simulink model "ProcessFlowRateModel_symbiotic"  (Simulink 7.9)
settings: Solver=VariableStepDiscrete  StartTime=0.0  StopTime=5000  RelTol=1e-3
libraries: simeventslib x11
settings Model: Creator=tsprock3  LastModifiedBy=tsprock3
settings DebuggingCC: SimStateOlderReleaseMsg=warning

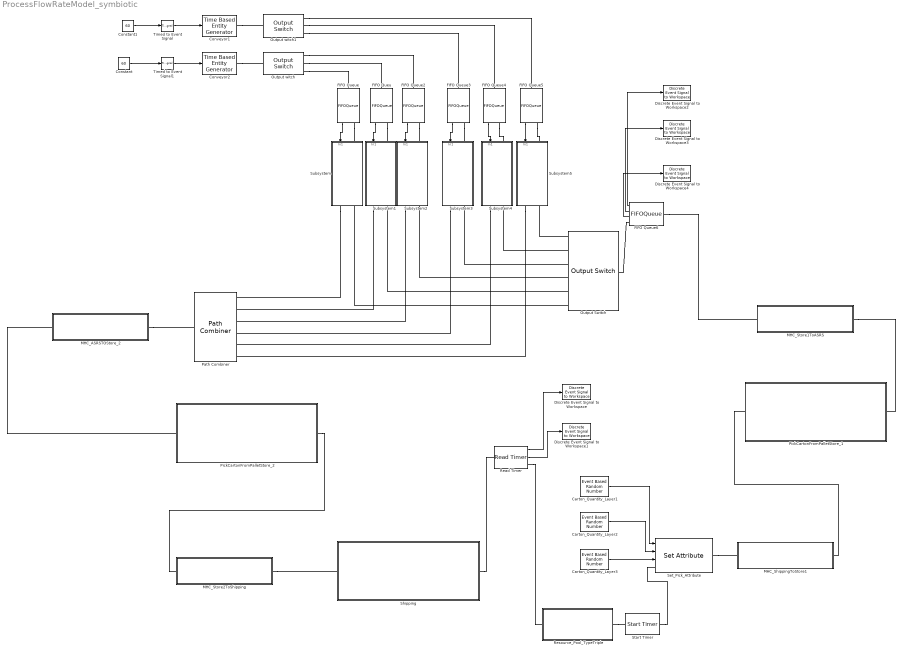
== system ProcessFlowRateModel_symbiotic ==
  Carton_Quantity_Layer1 : EventBasedRandomNumber  Distribution=Discrete uniform  minUnid=17  maxUnid=23  numValueUnid=7  valueVecDisc=[1 2 3]  probVecDisc=[0.5 0.35 0.15]  Seed=35621
  Carton_Quantity_Layer2 : EventBasedRandomNumber  Distribution=Discrete uniform  minUnid=55  maxUnid=65  numValueUnid=11  valueVecDisc=[1 2 3]  probVecDisc=[0.5 0.35 0.15]  Seed=38838
  Carton_Quantity_Layer3 : EventBasedRandomNumber  Distribution=Discrete uniform  minUnid=17  maxUnid=23  numValueUnid=7  valueVecDisc=[1 2 3]  probVecDisc=[0.5 0.35 0.15]  Seed=42055
  Constant : Constant  Value=60
  Constant1 : Constant  Value=60
  Conveyor1 : TimeBasedEntityGenerator  GenerateEntitiesUpon=Intergeneration time from port t
  Conveyor2 : TimeBasedEntityGenerator  GenerateEntitiesUpon=Intergeneration time from port t
  Discrete Event Signal to Workspace : simeventslib/SimEvents Sinks/Discrete Event Signal to Workspace  VariableName=elapsedtime  SaveFormat=Structure With Time  isMonitorOnly=off  isRecordIC=off
  Discrete Event Signal to Workspace1 : simeventslib/SimEvents Sinks/Discrete Event Signal to Workspace  VariableName=avg  SaveFormat=Structure With Time  isMonitorOnly=off  isRecordIC=off
  Discrete Event Signal to Workspace2 : simeventslib/SimEvents Sinks/Discrete Event Signal to Workspace  VariableName=serviced_qty  SaveFormat=Structure With Time  isMonitorOnly=off  isRecordIC=off
  Discrete Event Signal to Workspace3 : simeventslib/SimEvents Sinks/Discrete Event Signal to Workspace  VariableName=num_wait  SaveFormat=Structure With Time  isMonitorOnly=off  isRecordIC=off
  Discrete Event Signal to Workspace4 : simeventslib/SimEvents Sinks/Discrete Event Signal to Workspace  VariableName=avg_wait  SaveFormat=Structure With Time  isMonitorOnly=off  isRecordIC=off
  FIFO Queu : FIFOQueue  Capacity=1  StatNumberInBlock=on
      settings: OutputPortMap=o1
  FIFO Queue{,2..5} (5 alike) : FIFOQueue  Capacity=1  StatNumberInBlock=on
      settings: OutputPortMap=o1
  FIFO Queue6 : FIFOQueue  StatNumberDeparted=on  StatNumberInBlock=on  StatAverageWait=on
      settings: OutputPortMap=o0,o1,o2
  MHC_ASRSTOStore_2 : Subsystem
  MHC_ShippingToStore1 : Subsystem
  MHC_Store1ToASRS : Subsystem
  MHC_Store2ToShipping : Subsystem
  Output Switch : OutputSwitch  NumberOutputPorts=6
  Output witch : OutputSwitch  SwitchingCriterion=Round robin
  Output witch1 : OutputSwitch  SwitchingCriterion=Round robin
  Path Combiner : PathCombiner  NumberInputPorts=6
  PickCartonFromPalletStore_1 : Subsystem
  PickCartonFromPalletStore_2 : Subsystem
  Read Timer : ReadTimer  StatTimeElapsed=on  StatAverageTimeElapsed=on
      settings: OutputPortMap=o2,o3
  Resource_Pool_TypeTriple : Subsystem  mask{Quantity=33}
      mask prompts: Quantity "How many entities in resource pool?"
  Set_Pick_Attribute : SetAttribute  AttributeName=Carton_Quantity_Layer1|Carton_Quantity_Layer2|Carton_Quantity_Layer3  AttributeFrom=Signal port|Signal port|Signal port  AttributeValue=1|1|1  AttributeTreatAsVector=1|1|1  EvaluatedAttributeValue={[];[];[]}
      settings: InputPortMap=u0,u1,u2
  Shipping : Subsystem
  Start Timer : StartTimer  TimerStartedOption=Restart
  Subsystem : Subsystem
  Subsystem1 : Subsystem
  Subsystem2 : Subsystem
  Subsystem3 : Subsystem
  Subsystem4 : Subsystem
  Subsystem5 : Subsystem
  Timed to Event Signal : TimedToEventSignal
  Timed to Event Signal1 : TimedToEventSignal
  wires:
  Read Timer/1 -> Discrete Event Signal to Workspace/1
  Read Timer/2 -> Discrete Event Signal to Workspace1/1
  Carton_Quantity_Layer1/1 -> Set_Pick_Attribute/1
  Carton_Quantity_Layer2/1 -> Set_Pick_Attribute/2
  Carton_Quantity_Layer3/1 -> Set_Pick_Attribute/3
  FIFO Queue6/3 -> Discrete Event Signal to Workspace4/1
  FIFO Queue6/2 -> Discrete Event Signal to Workspace3/1
  FIFO Queue6/1 -> Discrete Event Signal to Workspace2/1
  Constant1/1 -> Timed to Event Signal/1
  Timed to Event Signal/1 -> Conveyor1/1
  Constant/1 -> Timed to Event Signal1/1
  Timed to Event Signal1/1 -> Conveyor2/1
  FIFO Queue/1 -> Subsystem/1(In1)
  FIFO Queu/1 -> Subsystem1/1(In1)
  FIFO Queue2/1 -> Subsystem2/1(In1)
  FIFO Queue3/1 -> Subsystem3/1(In1)
  FIFO Queue4/1 -> Subsystem4/1(In1)
  FIFO Queue5/1 -> Subsystem5/1(In1)
  connections:
  Set_Pick_Attribute/RConn1 -- MHC_ShippingToStore1/LConn1
  MHC_Store2ToShipping/RConn1 -- Shipping/LConn1
  MHC_ShippingToStore1/RConn1 -- PickCartonFromPalletStore_1/LConn1
  MHC_Store1ToASRS/LConn1 -- PickCartonFromPalletStore_1/RConn1
  PickCartonFromPalletStore_2/RConn1 -- MHC_Store2ToShipping/LConn1
  MHC_ASRSTOStore_2/RConn1 -- PickCartonFromPalletStore_2/LConn1
  Conveyor2/RConn1 -- Output witch/LConn1
  Output witch/RConn3 -- FIFO Queue/LConn1
  Output witch/RConn2 -- FIFO Queu/LConn1
  Output witch/RConn1 -- FIFO Queue2/LConn1
  Conveyor1/RConn1 -- Output witch1/LConn1
  Output witch1/RConn1 -- FIFO Queue5/LConn1
  Output witch1/RConn2 -- FIFO Queue4/LConn1
  Output witch1/RConn3 -- FIFO Queue3/LConn1
  FIFO Queue6/LConn1 -- MHC_Store1ToASRS/RConn1
  Shipping/RConn1 -- Read Timer/LConn1
  Resource_Pool_TypeTriple/LConn1 -- Start Timer/LConn1
  Start Timer/RConn1 -- Set_Pick_Attribute/LConn1
  Read Timer/RConn1 -- Resource_Pool_TypeTriple/RConn1
  FIFO Queue/RConn1 -- Subsystem/LConn1
  FIFO Queu/RConn1 -- Subsystem1/LConn1
  FIFO Queue2/RConn1 -- Subsystem2/LConn1
  FIFO Queue3/RConn1 -- Subsystem3/LConn1
  FIFO Queue4/RConn1 -- Subsystem4/LConn1
  FIFO Queue5/RConn1 -- Subsystem5/LConn1
  MHC_ASRSTOStore_2/LConn1 -- Path Combiner/RConn1
  Output Switch/LConn1 -- FIFO Queue6/RConn1
  Output Switch/RConn1 -- Subsystem5/RConn2
  Output Switch/RConn2 -- Subsystem4/RConn2
  Output Switch/RConn3 -- Subsystem3/RConn2
  Output Switch/RConn4 -- Subsystem2/RConn2
  Output Switch/RConn5 -- Subsystem1/RConn2
  Output Switch/RConn6 -- Subsystem/RConn2
  Subsystem/RConn1 -- Path Combiner/LConn1
  Subsystem1/RConn1 -- Path Combiner/LConn2
  Subsystem2/RConn1 -- Path Combiner/LConn3
  Subsystem3/RConn1 -- Path Combiner/LConn4
  Subsystem4/RConn1 -- Path Combiner/LConn5
  Subsystem5/RConn1 -- Path Combiner/LConn6

== system ProcessFlowRateModel_symbiotic/MHC_ASRSTOStore_2 ==
  note: This level provides an interface to access the Transportation_Channel block variant. The interface provides a method to
      | bring shipments in and route shipments out, as well as a consistent method to add ports to realize that interface
  IN_Shipment : PathCombiner  NumberInputPorts=1
  OUT_Shipment : OutputSwitch  NumberOutputPorts=1  AttributeName=Customer
  Transportation_Channel : Subsystem
  IN_Shipment_1 : PMIOPort  Port=1  Side=Left
  OUT_Shipment_1 : PMIOPort  Port=2  Side=Right
  connections:
  IN_Shipment/RConn1 -- Transportation_Channel/LConn1
  Transportation_Channel/RConn1 -- OUT_Shipment/LConn1
  IN_Shipment_1/RConn1 -- IN_Shipment/LConn1
  OUT_Shipment/RConn1 -- OUT_Shipment_1/RConn1

== system ProcessFlowRateModel_symbiotic/MHC_ShippingToStore1 ==
  note: This level provides an interface to access the Transportation_Channel block variant. The interface provides a method to
      | bring shipments in and route shipments out, as well as a consistent method to add ports to realize that interface
  IN_Shipment : PathCombiner  NumberInputPorts=1
  OUT_Shipment : OutputSwitch  NumberOutputPorts=1  AttributeName=Customer
  Transportation_Channel : Subsystem
  IN_Shipment_1 : PMIOPort  Port=1  Side=Left
  OUT_Shipment_1 : PMIOPort  Port=2  Side=Right
  connections:
  IN_Shipment/RConn1 -- Transportation_Channel/LConn1
  Transportation_Channel/RConn1 -- OUT_Shipment/LConn1
  IN_Shipment_1/RConn1 -- IN_Shipment/LConn1
  OUT_Shipment/RConn1 -- OUT_Shipment_1/RConn1

== system ProcessFlowRateModel_symbiotic/MHC_Store1ToASRS ==
  note: This level provides an interface to access the Transportation_Channel block variant. The interface provides a method to
      | bring shipments in and route shipments out, as well as a consistent method to add ports to realize that interface
  IN_Shipment : PathCombiner  NumberInputPorts=1
  OUT_Shipment : OutputSwitch  NumberOutputPorts=1  AttributeName=Customer
  Transportation_Channel : Subsystem
  IN_Shipment_1 : PMIOPort  Port=1  Side=Left
  OUT_Shipment_1 : PMIOPort  Port=2  Side=Right
  connections:
  IN_Shipment/RConn1 -- Transportation_Channel/LConn1
  Transportation_Channel/RConn1 -- OUT_Shipment/LConn1
  IN_Shipment_1/RConn1 -- IN_Shipment/LConn1
  OUT_Shipment/RConn1 -- OUT_Shipment_1/RConn1

== system ProcessFlowRateModel_symbiotic/MHC_Store2ToShipping ==
  note: This level provides an interface to access the Transportation_Channel block variant. The interface provides a method to
      | bring shipments in and route shipments out, as well as a consistent method to add ports to realize that interface
  IN_Shipment : PathCombiner  NumberInputPorts=1
  OUT_Shipment : OutputSwitch  NumberOutputPorts=1  AttributeName=Customer
  Transportation_Channel : Subsystem
  IN_Shipment_1 : PMIOPort  Port=1  Side=Left
  OUT_Shipment_1 : PMIOPort  Port=2  Side=Right
  connections:
  IN_Shipment/RConn1 -- Transportation_Channel/LConn1
  Transportation_Channel/RConn1 -- OUT_Shipment/LConn1
  IN_Shipment_1/RConn1 -- IN_Shipment/LConn1
  OUT_Shipment/RConn1 -- OUT_Shipment_1/RConn1

== system ProcessFlowRateModel_symbiotic/PickCartonFromPalletStore_1 ==
  IN_Job : PathCombiner  NumberInputPorts=1
  OUT_Job : OutputSwitch  NumberOutputPorts=1  SwitchingCriterion=Equiprobable  InitialSeed=9514
  Workstation : Subsystem
  IN_Job_1 : PMIOPort  Port=1  Side=Left
  OUT_Job_1 : PMIOPort  Port=2  Side=Right
  connections:
  IN_Job/RConn1 -- Workstation/LConn1
  Workstation/RConn1 -- OUT_Job/LConn1
  IN_Job_1/RConn1 -- IN_Job/LConn1
  OUT_Job/RConn1 -- OUT_Job_1/RConn1

== system ProcessFlowRateModel_symbiotic/PickCartonFromPalletStore_2 ==
  IN_Job : PathCombiner  NumberInputPorts=1
  OUT_Job : OutputSwitch  NumberOutputPorts=1  SwitchingCriterion=Equiprobable  InitialSeed=12731
  Workstation : Subsystem
  IN_Job_1 : PMIOPort  Port=1  Side=Left
  OUT_Job_1 : PMIOPort  Port=2  Side=Right
  connections:
  IN_Job/RConn1 -- Workstation/LConn1
  Workstation/RConn1 -- OUT_Job/LConn1
  IN_Job_1/RConn1 -- IN_Job/LConn1
  OUT_Job/RConn1 -- OUT_Job_1/RConn1

== system ProcessFlowRateModel_symbiotic/Resource_Pool_TypeTriple ==
  Event-Based Entity Generator : EventBasedEntityGenerator  GenerateEntitiesUpon=Function call from port fcn
  FIFO Queue : FIFOQueue  Capacity=inf
  FIFO Queue1 : FIFOQueue  Capacity=inf
  Path Combiner : PathCombiner  NumberInputPorts=2
  Release Gate : ReleaseGate  OpenGateUpon=Function call from port fcn
  Time-Based Function-Call Generator : TimeBasedFunctionCallGenerator  EventGenerationMode=Only at simulation start  NumberOfEventsPerPeriod=Quantity
  Time-Based Function-Call Generator1 : TimeBasedFunctionCallGenerator
  Acquire : PMIOPort  Port=1  Side=Left
  Return : PMIOPort  Port=2  Side=Right
  wires:
  Time-Based Function-Call Generator/1 -> Event-Based Entity Generator/1
  Time-Based Function-Call Generator1/1 -> Release Gate/1
  connections:
  Path Combiner/RConn1 -- FIFO Queue/LConn1
  Return/RConn1 -- Path Combiner/LConn2
  Acquire/RConn1 -- FIFO Queue/RConn1
  Event-Based Entity Generator/RConn1 -- FIFO Queue1/LConn1
  Release Gate/RConn1 -- Path Combiner/LConn1
  FIFO Queue1/RConn1 -- Release Gate/LConn1

== system ProcessFlowRateModel_symbiotic/Shipping ==
  IN_Job : PathCombiner  NumberInputPorts=1
  OUT_Job : OutputSwitch  NumberOutputPorts=1  SwitchingCriterion=Equiprobable  InitialSeed=15948
  Workstation : Subsystem
  IN_Job_1 : PMIOPort  Port=1  Side=Left
  OUT_Job_1 : PMIOPort  Port=2  Side=Right
  connections:
  IN_Job/RConn1 -- Workstation/LConn1
  Workstation/RConn1 -- OUT_Job/LConn1
  IN_Job_1/RConn1 -- IN_Job/LConn1
  OUT_Job/RConn1 -- OUT_Job_1/RConn1

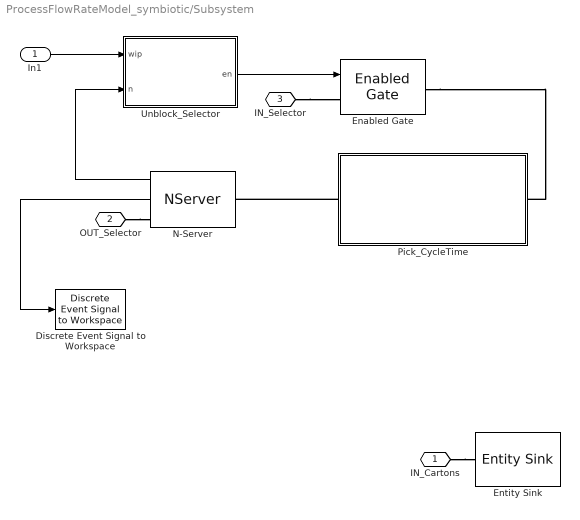
== system ProcessFlowRateModel_symbiotic/Subsystem ==
  In1 : Inport
  Discrete Event Signal to Workspace : simeventslib/SimEvents Sinks/Discrete Event Signal to Workspace  VariableName=utilization  SaveFormat=Structure With Time  isMonitorOnly=off  isRecordIC=off
  Enabled Gate : EnabledGate
  Entity Sink : EntitySink
  N-Server : NServer  NumberOfServers=1  ServiceTimeFrom=Attribute  ServiceTime=0  AttributeName=PickCycleTime  StatNumberInBlock=on  StatUtilization=on
      settings: OutputPortMap=o1,o5
  Pick_CycleTime : Subsystem  mask{pickmean=5, pickstddev=0.25, traveltime=0, qty=60}
      mask prompts: pickmean "eachPickMean"; pickstddev "eachPickStdDev"; qty "carton_qty"
  Unblock_Selector : Truth Table  TreatAsAtomicUnit=on
  IN_Cartons : PMIOPort  Port=1  Side=Left
  OUT_Selector : PMIOPort  Port=2  Side=Right
  IN_Selector : PMIOPort  Port=3  Side=Right
  wires:
  N-Server/2 -> Discrete Event Signal to Workspace/1
  In1/1 -> Unblock_Selector/1(wip)
  N-Server/1 -> Unblock_Selector/2(n)
  Unblock_Selector/1(en) -> Enabled Gate/1
  connections:
  Enabled Gate/RConn1 -- Pick_CycleTime/LConn1
  Pick_CycleTime/RConn1 -- N-Server/LConn1
  IN_Cartons/RConn1 -- Entity Sink/LConn1
  IN_Selector/RConn1 -- Enabled Gate/LConn1
  OUT_Selector/RConn1 -- N-Server/RConn1

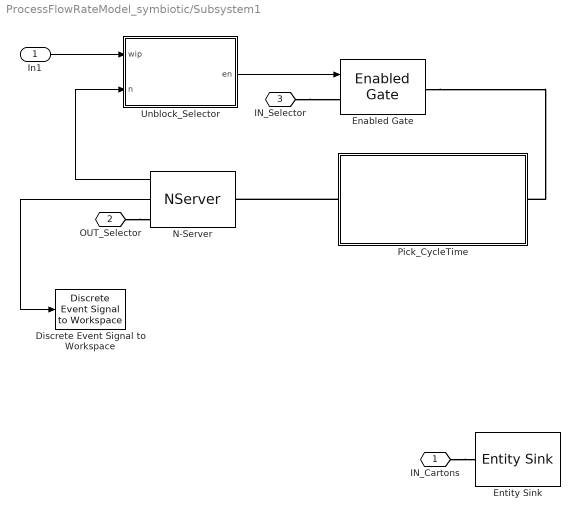
== system ProcessFlowRateModel_symbiotic/Subsystem1 ==
  In1 : Inport
  Discrete Event Signal to Workspace : simeventslib/SimEvents Sinks/Discrete Event Signal to Workspace  VariableName=utilization  SaveFormat=Structure With Time  isMonitorOnly=off  isRecordIC=off
  Enabled Gate : EnabledGate
  Entity Sink : EntitySink
  N-Server : NServer  NumberOfServers=1  ServiceTimeFrom=Attribute  ServiceTime=0  AttributeName=PickCycleTime  StatNumberInBlock=on  StatUtilization=on
      settings: OutputPortMap=o1,o5
  Pick_CycleTime : Subsystem  mask{pickmean=5, pickstddev=0.25, traveltime=0, qty=60}
      mask prompts: pickmean "eachPickMean"; pickstddev "eachPickStdDev"; qty "carton_qty"
  Unblock_Selector : Truth Table  TreatAsAtomicUnit=on
  IN_Cartons : PMIOPort  Port=1  Side=Left
  OUT_Selector : PMIOPort  Port=2  Side=Right
  IN_Selector : PMIOPort  Port=3  Side=Right
  wires:
  N-Server/2 -> Discrete Event Signal to Workspace/1
  In1/1 -> Unblock_Selector/1(wip)
  N-Server/1 -> Unblock_Selector/2(n)
  Unblock_Selector/1(en) -> Enabled Gate/1
  connections:
  Enabled Gate/RConn1 -- Pick_CycleTime/LConn1
  Pick_CycleTime/RConn1 -- N-Server/LConn1
  IN_Cartons/RConn1 -- Entity Sink/LConn1
  IN_Selector/RConn1 -- Enabled Gate/LConn1
  OUT_Selector/RConn1 -- N-Server/RConn1

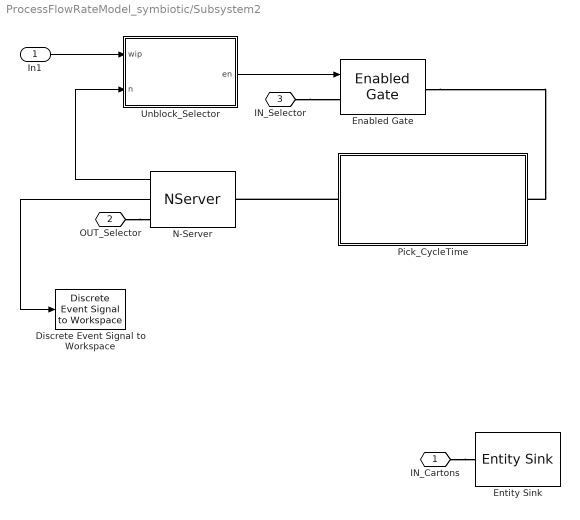
== system ProcessFlowRateModel_symbiotic/Subsystem2 ==
  In1 : Inport
  Discrete Event Signal to Workspace : simeventslib/SimEvents Sinks/Discrete Event Signal to Workspace  VariableName=utilization  SaveFormat=Structure With Time  isMonitorOnly=off  isRecordIC=off
  Enabled Gate : EnabledGate
  Entity Sink : EntitySink
  N-Server : NServer  NumberOfServers=1  ServiceTimeFrom=Attribute  ServiceTime=0  AttributeName=PickCycleTime  StatNumberInBlock=on  StatUtilization=on
      settings: OutputPortMap=o1,o5
  Pick_CycleTime : Subsystem  mask{pickmean=5, pickstddev=0.25, traveltime=0, qty=60}
      mask prompts: pickmean "eachPickMean"; pickstddev "eachPickStdDev"; qty "carton_qty"
  Unblock_Selector : Truth Table  TreatAsAtomicUnit=on
  IN_Cartons : PMIOPort  Port=1  Side=Left
  OUT_Selector : PMIOPort  Port=2  Side=Right
  IN_Selector : PMIOPort  Port=3  Side=Right
  wires:
  N-Server/2 -> Discrete Event Signal to Workspace/1
  In1/1 -> Unblock_Selector/1(wip)
  N-Server/1 -> Unblock_Selector/2(n)
  Unblock_Selector/1(en) -> Enabled Gate/1
  connections:
  Enabled Gate/RConn1 -- Pick_CycleTime/LConn1
  Pick_CycleTime/RConn1 -- N-Server/LConn1
  IN_Cartons/RConn1 -- Entity Sink/LConn1
  IN_Selector/RConn1 -- Enabled Gate/LConn1
  OUT_Selector/RConn1 -- N-Server/RConn1

== system ProcessFlowRateModel_symbiotic/Subsystem3 ==
  In1 : Inport
  Discrete Event Signal to Workspace : simeventslib/SimEvents Sinks/Discrete Event Signal to Workspace  VariableName=utilization  SaveFormat=Structure With Time  isMonitorOnly=off  isRecordIC=off
  Enabled Gate : EnabledGate
  Entity Sink : EntitySink
  N-Server : NServer  NumberOfServers=1  ServiceTimeFrom=Attribute  ServiceTime=0  AttributeName=PickCycleTime  StatNumberInBlock=on  StatUtilization=on
      settings: OutputPortMap=o1,o5
  Pick_CycleTime : Subsystem  mask{pickmean=5, pickstddev=0.25, traveltime=0, qty=60}
      mask prompts: pickmean "eachPickMean"; pickstddev "eachPickStdDev"; qty "carton_qty"
  Unblock_Selector : Truth Table  TreatAsAtomicUnit=on
  IN_Cartons : PMIOPort  Port=1  Side=Left
  OUT_Selector : PMIOPort  Port=2  Side=Right
  IN_Selector : PMIOPort  Port=3  Side=Right
  wires:
  N-Server/2 -> Discrete Event Signal to Workspace/1
  In1/1 -> Unblock_Selector/1(wip)
  N-Server/1 -> Unblock_Selector/2(n)
  Unblock_Selector/1(en) -> Enabled Gate/1
  connections:
  Enabled Gate/RConn1 -- Pick_CycleTime/LConn1
  Pick_CycleTime/RConn1 -- N-Server/LConn1
  IN_Cartons/RConn1 -- Entity Sink/LConn1
  IN_Selector/RConn1 -- Enabled Gate/LConn1
  OUT_Selector/RConn1 -- N-Server/RConn1

== system ProcessFlowRateModel_symbiotic/Subsystem4 ==
  In1 : Inport
  Discrete Event Signal to Workspace : simeventslib/SimEvents Sinks/Discrete Event Signal to Workspace  VariableName=utilization  SaveFormat=Structure With Time  isMonitorOnly=off  isRecordIC=off
  Enabled Gate : EnabledGate
  Entity Sink : EntitySink
  N-Server : NServer  NumberOfServers=1  ServiceTimeFrom=Attribute  ServiceTime=0  AttributeName=PickCycleTime  StatNumberInBlock=on  StatUtilization=on
      settings: OutputPortMap=o1,o5
  Pick_CycleTime : Subsystem  mask{pickmean=5, pickstddev=0.25, traveltime=0, qty=60}
      mask prompts: pickmean "eachPickMean"; pickstddev "eachPickStdDev"; qty "carton_qty"
  Unblock_Selector : Truth Table  TreatAsAtomicUnit=on
  IN_Cartons : PMIOPort  Port=1  Side=Left
  OUT_Selector : PMIOPort  Port=2  Side=Right
  IN_Selector : PMIOPort  Port=3  Side=Right
  wires:
  N-Server/2 -> Discrete Event Signal to Workspace/1
  In1/1 -> Unblock_Selector/1(wip)
  N-Server/1 -> Unblock_Selector/2(n)
  Unblock_Selector/1(en) -> Enabled Gate/1
  connections:
  Enabled Gate/RConn1 -- Pick_CycleTime/LConn1
  Pick_CycleTime/RConn1 -- N-Server/LConn1
  IN_Cartons/RConn1 -- Entity Sink/LConn1
  IN_Selector/RConn1 -- Enabled Gate/LConn1
  OUT_Selector/RConn1 -- N-Server/RConn1

== system ProcessFlowRateModel_symbiotic/Subsystem5 ==
  In1 : Inport
  Discrete Event Signal to Workspace : simeventslib/SimEvents Sinks/Discrete Event Signal to Workspace  VariableName=utilization  SaveFormat=Structure With Time  isMonitorOnly=off  isRecordIC=off
  Enabled Gate : EnabledGate
  Entity Sink : EntitySink
  N-Server : NServer  NumberOfServers=1  ServiceTimeFrom=Attribute  ServiceTime=0  AttributeName=PickCycleTime  StatNumberInBlock=on  StatUtilization=on
      settings: OutputPortMap=o1,o5
  Pick_CycleTime : Subsystem  mask{pickmean=5, pickstddev=0.25, traveltime=0, qty=60}
      mask prompts: pickmean "eachPickMean"; pickstddev "eachPickStdDev"; qty "carton_qty"
  Unblock_Selector : Truth Table  TreatAsAtomicUnit=on
  IN_Cartons : PMIOPort  Port=1  Side=Left
  OUT_Selector : PMIOPort  Port=2  Side=Right
  IN_Selector : PMIOPort  Port=3  Side=Right
  wires:
  N-Server/2 -> Discrete Event Signal to Workspace/1
  In1/1 -> Unblock_Selector/1(wip)
  N-Server/1 -> Unblock_Selector/2(n)
  Unblock_Selector/1(en) -> Enabled Gate/1
  connections:
  Enabled Gate/RConn1 -- Pick_CycleTime/LConn1
  Pick_CycleTime/RConn1 -- N-Server/LConn1
  IN_Cartons/RConn1 -- Entity Sink/LConn1
  IN_Selector/RConn1 -- Enabled Gate/LConn1
  OUT_Selector/RConn1 -- N-Server/RConn1

== system ProcessFlowRateModel_symbiotic/MHC_ASRSTOStore_2/Transportation_Channel ==
  FIFO Queue : FIFOQueue  Capacity=inf
  N-Server : NServer  NumberOfServers=inf  ServiceTime=10
  IN_Shipment : PMIOPort  Port=1  Side=Left
  OUT_Shipment : PMIOPort  Port=2  Side=Right
  connections:
  FIFO Queue/RConn1 -- N-Server/LConn1
  IN_Shipment/RConn1 -- FIFO Queue/LConn1
  OUT_Shipment/RConn1 -- N-Server/RConn1

== system ProcessFlowRateModel_symbiotic/MHC_ShippingToStore1/Transportation_Channel ==
  FIFO Queue : FIFOQueue  Capacity=inf
  N-Server : NServer  NumberOfServers=inf  ServiceTime=20
  IN_Shipment : PMIOPort  Port=1  Side=Left
  OUT_Shipment : PMIOPort  Port=2  Side=Right
  connections:
  FIFO Queue/RConn1 -- N-Server/LConn1
  IN_Shipment/RConn1 -- FIFO Queue/LConn1
  OUT_Shipment/RConn1 -- N-Server/RConn1

== system ProcessFlowRateModel_symbiotic/MHC_Store1ToASRS/Transportation_Channel ==
  FIFO Queue : FIFOQueue  Capacity=inf
  N-Server : NServer  NumberOfServers=inf  ServiceTime=10
  IN_Shipment : PMIOPort  Port=1  Side=Left
  OUT_Shipment : PMIOPort  Port=2  Side=Right
  connections:
  FIFO Queue/RConn1 -- N-Server/LConn1
  IN_Shipment/RConn1 -- FIFO Queue/LConn1
  OUT_Shipment/RConn1 -- N-Server/RConn1

== system ProcessFlowRateModel_symbiotic/MHC_Store2ToShipping/Transportation_Channel ==
  FIFO Queue : FIFOQueue  Capacity=inf
  N-Server : NServer  NumberOfServers=inf  ServiceTime=20
  IN_Shipment : PMIOPort  Port=1  Side=Left
  OUT_Shipment : PMIOPort  Port=2  Side=Right
  connections:
  FIFO Queue/RConn1 -- N-Server/LConn1
  IN_Shipment/RConn1 -- FIFO Queue/LConn1
  OUT_Shipment/RConn1 -- N-Server/RConn1

== system ProcessFlowRateModel_symbiotic/PickCartonFromPalletStore_1/Workstation ==
  CartonPick : Subsystem
  Entity_Combiner : EntityCombiner  NumberInputPorts=1
  Entity_Splitter : EntitySplitter  NumberOutputPorts=1
  FIFO Queue : FIFOQueue
  OUT_Job_1 : PMIOPort  Port=1  Side=Right
  IN_Job_1 : PMIOPort  Port=2  Side=Left
  connections:
  FIFO Queue/RConn1 -- Entity_Combiner/LConn1
  Entity_Splitter/RConn1 -- OUT_Job_1/RConn1
  IN_Job_1/RConn1 -- FIFO Queue/LConn1
  Entity_Combiner/RConn1 -- CartonPick/LConn1
  CartonPick/RConn1 -- Entity_Splitter/LConn1

== system ProcessFlowRateModel_symbiotic/PickCartonFromPalletStore_2/Workstation ==
  CartonPick : Subsystem
  Entity_Combiner : EntityCombiner  NumberInputPorts=1
  Entity_Splitter : EntitySplitter  NumberOutputPorts=1
  FIFO Queue : FIFOQueue
  OUT_Job_1 : PMIOPort  Port=1  Side=Right
  IN_Job_1 : PMIOPort  Port=2  Side=Left
  connections:
  FIFO Queue/RConn1 -- Entity_Combiner/LConn1
  Entity_Splitter/RConn1 -- OUT_Job_1/RConn1
  IN_Job_1/RConn1 -- FIFO Queue/LConn1
  Entity_Combiner/RConn1 -- CartonPick/LConn1
  CartonPick/RConn1 -- Entity_Splitter/LConn1

== system ProcessFlowRateModel_symbiotic/Shipping/Workstation ==
  Entity_Combiner : EntityCombiner  NumberInputPorts=1
  Entity_Splitter : EntitySplitter  NumberOutputPorts=1
  FIFO Queue : FIFOQueue
  Shipping : Subsystem
  OUT_Job_1 : PMIOPort  Port=1  Side=Right
  IN_Job_1 : PMIOPort  Port=2  Side=Left
  connections:
  FIFO Queue/RConn1 -- Entity_Combiner/LConn1
  Entity_Splitter/RConn1 -- OUT_Job_1/RConn1
  IN_Job_1/RConn1 -- FIFO Queue/LConn1
  Entity_Combiner/RConn1 -- Shipping/LConn1
  Shipping/RConn1 -- Entity_Splitter/LConn1

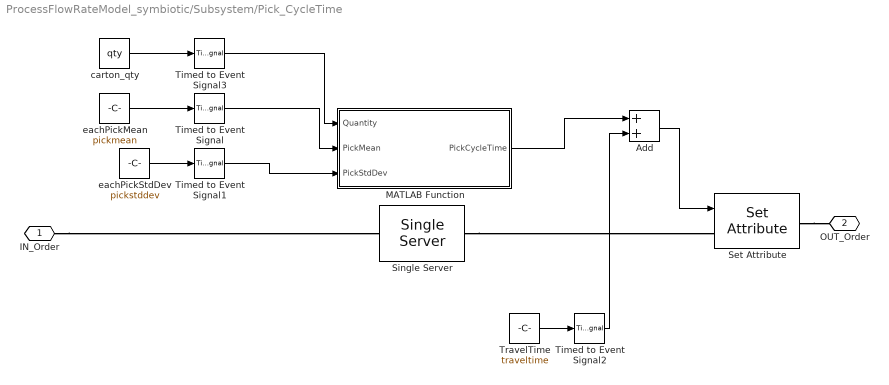
== system ProcessFlowRateModel_symbiotic/Subsystem/Pick_CycleTime ==
  Add : Sum
  MATLAB Function : MATLAB Function  TreatAsAtomicUnit=on
  Set Attribute : SetAttribute  AttributeName=PickCycleTime  AttributeFrom=Signal port  EvaluatedAttributeValue={[]}
  Single Server : SingleServer  ServiceTime=0
  Timed to Event Signal{,1..3} (4 alike) : TimedToEventSignal
  TravelTime : Constant  Value=traveltime
  carton_qty : Constant  Value=qty
  eachPickMean : Constant  Value=pickmean
  eachPickStdDev : Constant  Value=pickstddev
  IN_Order : PMIOPort  Port=1  Side=Left
  OUT_Order : PMIOPort  Port=2  Side=Right
  wires:
  MATLAB Function/1(PickCycleTime) -> Add/1
  eachPickStdDev/1 -> Timed to Event Signal1/1
  Timed to Event Signal1/1 -> MATLAB Function/3(PickStdDev)
  eachPickMean/1 -> Timed to Event Signal/1
  Timed to Event Signal/1 -> MATLAB Function/2(PickMean)
  TravelTime/1 -> Timed to Event Signal2/1
  Timed to Event Signal2/1 -> Add/2
  carton_qty/1 -> Timed to Event Signal3/1
  Timed to Event Signal3/1 -> MATLAB Function/1(Quantity)
  Add/1 -> Set Attribute/1
  connections:
  IN_Order/RConn1 -- Single Server/LConn1
  Set Attribute/RConn1 -- OUT_Order/RConn1
  Single Server/RConn1 -- Set Attribute/LConn1

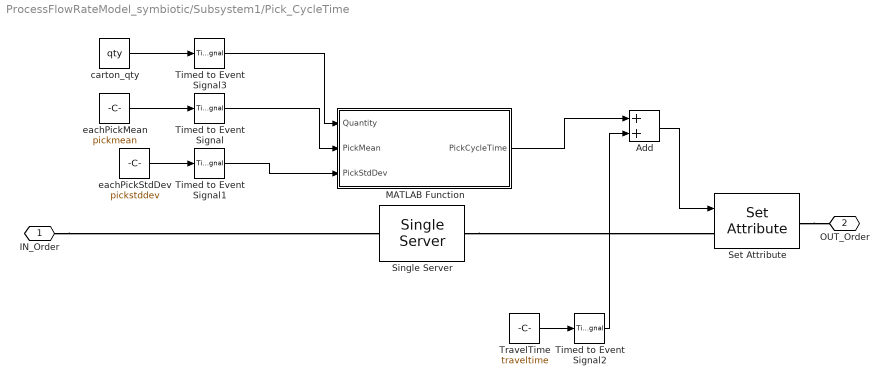
== system ProcessFlowRateModel_symbiotic/Subsystem1/Pick_CycleTime ==
  Add : Sum
  MATLAB Function : MATLAB Function  TreatAsAtomicUnit=on
  Set Attribute : SetAttribute  AttributeName=PickCycleTime  AttributeFrom=Signal port  EvaluatedAttributeValue={[]}
  Single Server : SingleServer  ServiceTime=0
  Timed to Event Signal{,1..3} (4 alike) : TimedToEventSignal
  TravelTime : Constant  Value=traveltime
  carton_qty : Constant  Value=qty
  eachPickMean : Constant  Value=pickmean
  eachPickStdDev : Constant  Value=pickstddev
  IN_Order : PMIOPort  Port=1  Side=Left
  OUT_Order : PMIOPort  Port=2  Side=Right
  wires:
  MATLAB Function/1(PickCycleTime) -> Add/1
  eachPickStdDev/1 -> Timed to Event Signal1/1
  Timed to Event Signal1/1 -> MATLAB Function/3(PickStdDev)
  eachPickMean/1 -> Timed to Event Signal/1
  Timed to Event Signal/1 -> MATLAB Function/2(PickMean)
  TravelTime/1 -> Timed to Event Signal2/1
  Timed to Event Signal2/1 -> Add/2
  carton_qty/1 -> Timed to Event Signal3/1
  Timed to Event Signal3/1 -> MATLAB Function/1(Quantity)
  Add/1 -> Set Attribute/1
  connections:
  IN_Order/RConn1 -- Single Server/LConn1
  Set Attribute/RConn1 -- OUT_Order/RConn1
  Single Server/RConn1 -- Set Attribute/LConn1

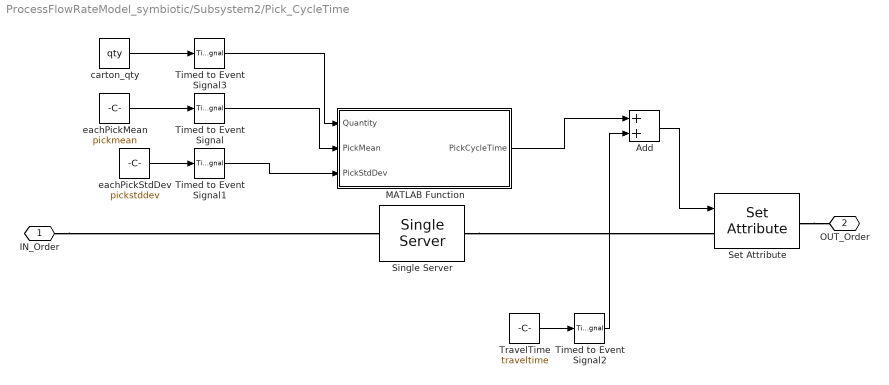
== system ProcessFlowRateModel_symbiotic/Subsystem2/Pick_CycleTime ==
  Add : Sum
  MATLAB Function : MATLAB Function  TreatAsAtomicUnit=on
  Set Attribute : SetAttribute  AttributeName=PickCycleTime  AttributeFrom=Signal port  EvaluatedAttributeValue={[]}
  Single Server : SingleServer  ServiceTime=0
  Timed to Event Signal{,1..3} (4 alike) : TimedToEventSignal
  TravelTime : Constant  Value=traveltime
  carton_qty : Constant  Value=qty
  eachPickMean : Constant  Value=pickmean
  eachPickStdDev : Constant  Value=pickstddev
  IN_Order : PMIOPort  Port=1  Side=Left
  OUT_Order : PMIOPort  Port=2  Side=Right
  wires:
  MATLAB Function/1(PickCycleTime) -> Add/1
  eachPickStdDev/1 -> Timed to Event Signal1/1
  Timed to Event Signal1/1 -> MATLAB Function/3(PickStdDev)
  eachPickMean/1 -> Timed to Event Signal/1
  Timed to Event Signal/1 -> MATLAB Function/2(PickMean)
  TravelTime/1 -> Timed to Event Signal2/1
  Timed to Event Signal2/1 -> Add/2
  carton_qty/1 -> Timed to Event Signal3/1
  Timed to Event Signal3/1 -> MATLAB Function/1(Quantity)
  Add/1 -> Set Attribute/1
  connections:
  IN_Order/RConn1 -- Single Server/LConn1
  Set Attribute/RConn1 -- OUT_Order/RConn1
  Single Server/RConn1 -- Set Attribute/LConn1

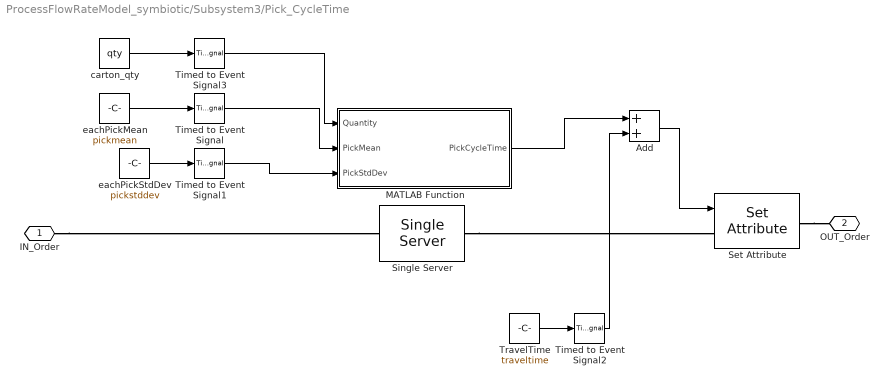
== system ProcessFlowRateModel_symbiotic/Subsystem3/Pick_CycleTime ==
  Add : Sum
  MATLAB Function : MATLAB Function  TreatAsAtomicUnit=on
  Set Attribute : SetAttribute  AttributeName=PickCycleTime  AttributeFrom=Signal port  EvaluatedAttributeValue={[]}
  Single Server : SingleServer  ServiceTime=0
  Timed to Event Signal{,1..3} (4 alike) : TimedToEventSignal
  TravelTime : Constant  Value=traveltime
  carton_qty : Constant  Value=qty
  eachPickMean : Constant  Value=pickmean
  eachPickStdDev : Constant  Value=pickstddev
  IN_Order : PMIOPort  Port=1  Side=Left
  OUT_Order : PMIOPort  Port=2  Side=Right
  wires:
  MATLAB Function/1(PickCycleTime) -> Add/1
  eachPickStdDev/1 -> Timed to Event Signal1/1
  Timed to Event Signal1/1 -> MATLAB Function/3(PickStdDev)
  eachPickMean/1 -> Timed to Event Signal/1
  Timed to Event Signal/1 -> MATLAB Function/2(PickMean)
  TravelTime/1 -> Timed to Event Signal2/1
  Timed to Event Signal2/1 -> Add/2
  carton_qty/1 -> Timed to Event Signal3/1
  Timed to Event Signal3/1 -> MATLAB Function/1(Quantity)
  Add/1 -> Set Attribute/1
  connections:
  IN_Order/RConn1 -- Single Server/LConn1
  Set Attribute/RConn1 -- OUT_Order/RConn1
  Single Server/RConn1 -- Set Attribute/LConn1

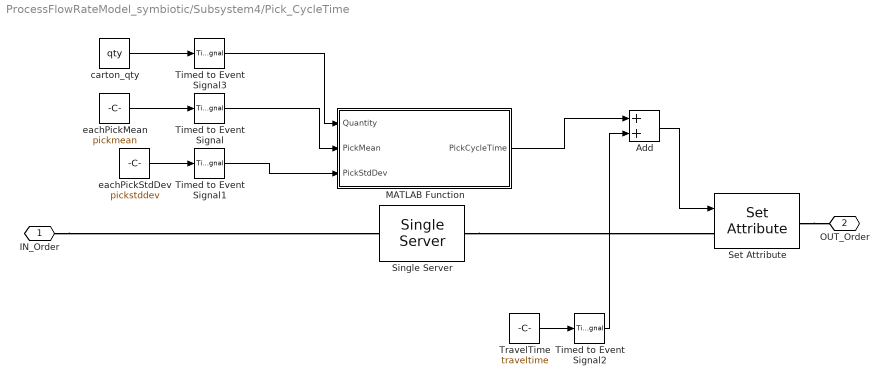
== system ProcessFlowRateModel_symbiotic/Subsystem4/Pick_CycleTime ==
  Add : Sum
  MATLAB Function : MATLAB Function  TreatAsAtomicUnit=on
  Set Attribute : SetAttribute  AttributeName=PickCycleTime  AttributeFrom=Signal port  EvaluatedAttributeValue={[]}
  Single Server : SingleServer  ServiceTime=0
  Timed to Event Signal{,1..3} (4 alike) : TimedToEventSignal
  TravelTime : Constant  Value=traveltime
  carton_qty : Constant  Value=qty
  eachPickMean : Constant  Value=pickmean
  eachPickStdDev : Constant  Value=pickstddev
  IN_Order : PMIOPort  Port=1  Side=Left
  OUT_Order : PMIOPort  Port=2  Side=Right
  wires:
  MATLAB Function/1(PickCycleTime) -> Add/1
  eachPickStdDev/1 -> Timed to Event Signal1/1
  Timed to Event Signal1/1 -> MATLAB Function/3(PickStdDev)
  eachPickMean/1 -> Timed to Event Signal/1
  Timed to Event Signal/1 -> MATLAB Function/2(PickMean)
  TravelTime/1 -> Timed to Event Signal2/1
  Timed to Event Signal2/1 -> Add/2
  carton_qty/1 -> Timed to Event Signal3/1
  Timed to Event Signal3/1 -> MATLAB Function/1(Quantity)
  Add/1 -> Set Attribute/1
  connections:
  IN_Order/RConn1 -- Single Server/LConn1
  Set Attribute/RConn1 -- OUT_Order/RConn1
  Single Server/RConn1 -- Set Attribute/LConn1

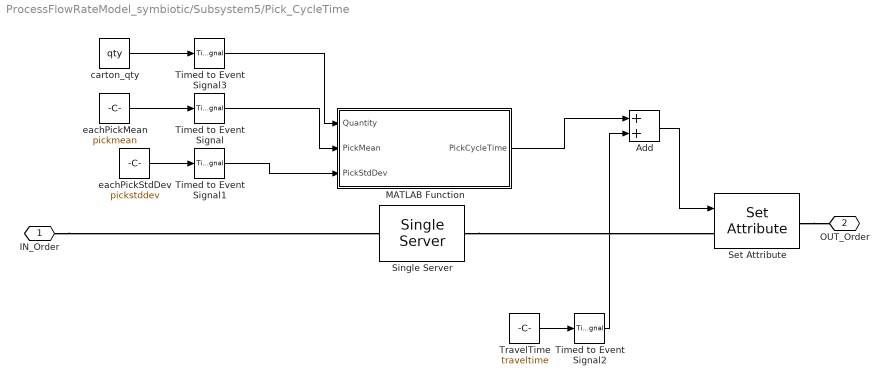
== system ProcessFlowRateModel_symbiotic/Subsystem5/Pick_CycleTime ==
  Add : Sum
  MATLAB Function : MATLAB Function  TreatAsAtomicUnit=on
  Set Attribute : SetAttribute  AttributeName=PickCycleTime  AttributeFrom=Signal port  EvaluatedAttributeValue={[]}
  Single Server : SingleServer  ServiceTime=0
  Timed to Event Signal{,1..3} (4 alike) : TimedToEventSignal
  TravelTime : Constant  Value=traveltime
  carton_qty : Constant  Value=qty
  eachPickMean : Constant  Value=pickmean
  eachPickStdDev : Constant  Value=pickstddev
  IN_Order : PMIOPort  Port=1  Side=Left
  OUT_Order : PMIOPort  Port=2  Side=Right
  wires:
  MATLAB Function/1(PickCycleTime) -> Add/1
  eachPickStdDev/1 -> Timed to Event Signal1/1
  Timed to Event Signal1/1 -> MATLAB Function/3(PickStdDev)
  eachPickMean/1 -> Timed to Event Signal/1
  Timed to Event Signal/1 -> MATLAB Function/2(PickMean)
  TravelTime/1 -> Timed to Event Signal2/1
  Timed to Event Signal2/1 -> Add/2
  carton_qty/1 -> Timed to Event Signal3/1
  Timed to Event Signal3/1 -> MATLAB Function/1(Quantity)
  Add/1 -> Set Attribute/1
  connections:
  IN_Order/RConn1 -- Single Server/LConn1
  Set Attribute/RConn1 -- OUT_Order/RConn1
  Single Server/RConn1 -- Set Attribute/LConn1

== system ProcessFlowRateModel_symbiotic/PickCartonFromPalletStore_1/Workstation/CartonPick ==
  FIFO Queue : FIFOQueue
  N-Server : NServer  NumberOfServers=inf  ServiceTimeFrom=Signal port t  ServiceTime=0
  Pick_CycleTime : Subsystem  mask{pickmean=5, pickstddev=0.25, traveltime=80}
      mask prompts: pickmean "eachPickMean"; pickstddev "eachPickStdDev"
  Flow_IN : PMIOPort  Port=1  Side=Left
  Message_IN : PMIOPort  Port=2  Side=Left
  Flow_OUT : PMIOPort  Port=3  Side=Right
  Message_OUT : PMIOPort  Port=4  Side=Right
  wires:
  Pick_CycleTime/1(PickCycleTime) -> N-Server/1
  connections:
  Flow_IN/RConn1 -- FIFO Queue/LConn1
  Flow_OUT/RConn1 -- N-Server/RConn1
  Message_OUT/RConn1 -- Message_IN/RConn1
  FIFO Queue/RConn1 -- Pick_CycleTime/LConn1
  Pick_CycleTime/RConn1 -- N-Server/LConn1

== system ProcessFlowRateModel_symbiotic/PickCartonFromPalletStore_2/Workstation/CartonPick ==
  FIFO Queue : FIFOQueue
  N-Server : NServer  NumberOfServers=inf  ServiceTimeFrom=Signal port t  ServiceTime=0
  Pick_CycleTime : Subsystem  mask{pickmean=5, pickstddev=0.25, traveltime=80}
      mask prompts: pickmean "eachPickMean"; pickstddev "eachPickStdDev"
  Flow_IN : PMIOPort  Port=1  Side=Left
  Message_IN : PMIOPort  Port=2  Side=Left
  Flow_OUT : PMIOPort  Port=3  Side=Right
  Message_OUT : PMIOPort  Port=4  Side=Right
  wires:
  Pick_CycleTime/1(PickCycleTime) -> N-Server/1
  connections:
  Flow_IN/RConn1 -- FIFO Queue/LConn1
  Flow_OUT/RConn1 -- N-Server/RConn1
  Message_OUT/RConn1 -- Message_IN/RConn1
  FIFO Queue/RConn1 -- Pick_CycleTime/LConn1
  Pick_CycleTime/RConn1 -- N-Server/LConn1

== system ProcessFlowRateModel_symbiotic/Shipping/Workstation/Shipping ==
  IN_Job : PathCombiner  NumberInputPorts=1
  OUT_Job : OutputSwitch  NumberOutputPorts=1  SwitchingCriterion=Equiprobable  InitialSeed=65399
  Process : Subsystem
  IN_Job_1 : PMIOPort  Port=1  Side=Left
  OUT_Job_1 : PMIOPort  Port=2  Side=Right
  connections:
  IN_Job/RConn1 -- Process/LConn1
  Process/RConn1 -- OUT_Job/LConn1
  IN_Job_1/RConn1 -- IN_Job/LConn1
  OUT_Job_1/RConn1 -- OUT_Job/RConn1

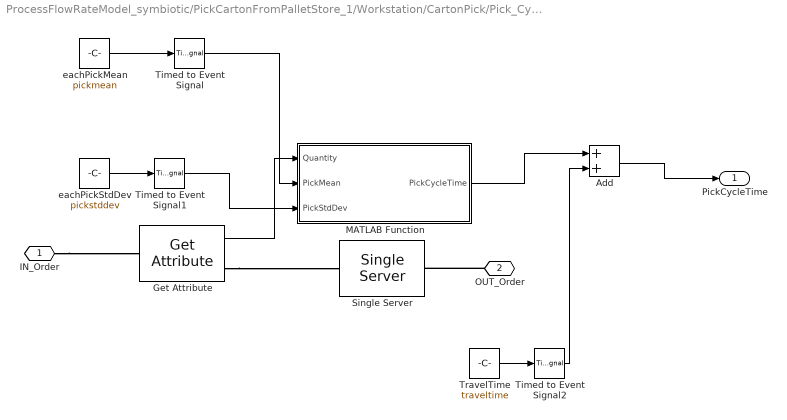
== system ProcessFlowRateModel_symbiotic/PickCartonFromPalletStore_1/Workstation/CartonPick/Pick_CycleTime ==
  Add : Sum
  Get Attribute : GetAttribute  AttributeName=Carton_Quantity_Layer1  EvaluatedDefaultAttributeValue={[]}
      settings: OutputPortMap=o1
  MATLAB Function : MATLAB Function  TreatAsAtomicUnit=on
  Single Server : SingleServer  ServiceTime=0
  Timed to Event Signal : TimedToEventSignal
  Timed to Event Signal1 : TimedToEventSignal
  Timed to Event Signal2 : TimedToEventSignal
  TravelTime : Constant  Value=traveltime
  eachPickMean : Constant  Value=pickmean
  eachPickStdDev : Constant  Value=pickstddev
  IN_Order : PMIOPort  Port=1  Side=Left
  OUT_Order : PMIOPort  Port=2  Side=Right
  PickCycleTime : Outport
  wires:
  Get Attribute/1 -> MATLAB Function/1(Quantity)
  MATLAB Function/1(PickCycleTime) -> Add/1
  Add/1 -> PickCycleTime/1
  eachPickStdDev/1 -> Timed to Event Signal1/1
  Timed to Event Signal1/1 -> MATLAB Function/3(PickStdDev)
  eachPickMean/1 -> Timed to Event Signal/1
  Timed to Event Signal/1 -> MATLAB Function/2(PickMean)
  TravelTime/1 -> Timed to Event Signal2/1
  Timed to Event Signal2/1 -> Add/2
  connections:
  Get Attribute/RConn1 -- Single Server/LConn1
  IN_Order/RConn1 -- Get Attribute/LConn1
  OUT_Order/RConn1 -- Single Server/RConn1

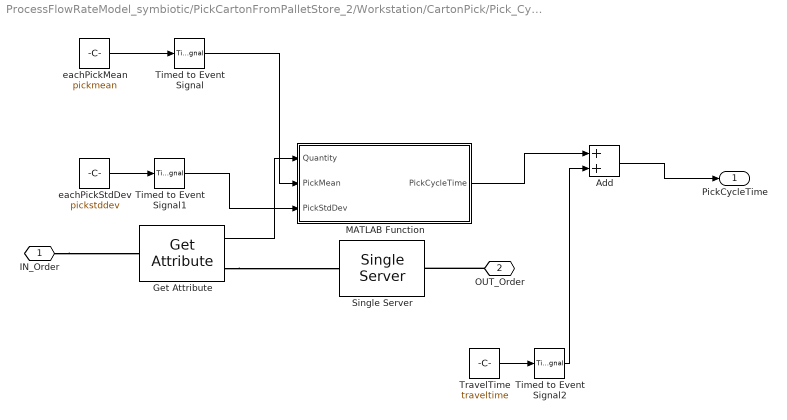
== system ProcessFlowRateModel_symbiotic/PickCartonFromPalletStore_2/Workstation/CartonPick/Pick_CycleTime ==
  Add : Sum
  Get Attribute : GetAttribute  AttributeName=Carton_Quantity_Layer3  EvaluatedDefaultAttributeValue={[]}
      settings: OutputPortMap=o1
  MATLAB Function : MATLAB Function  TreatAsAtomicUnit=on
  Single Server : SingleServer  ServiceTime=0
  Timed to Event Signal : TimedToEventSignal
  Timed to Event Signal1 : TimedToEventSignal
  Timed to Event Signal2 : TimedToEventSignal
  TravelTime : Constant  Value=traveltime
  eachPickMean : Constant  Value=pickmean
  eachPickStdDev : Constant  Value=pickstddev
  IN_Order : PMIOPort  Port=1  Side=Left
  OUT_Order : PMIOPort  Port=2  Side=Right
  PickCycleTime : Outport
  wires:
  Get Attribute/1 -> MATLAB Function/1(Quantity)
  MATLAB Function/1(PickCycleTime) -> Add/1
  Add/1 -> PickCycleTime/1
  eachPickStdDev/1 -> Timed to Event Signal1/1
  Timed to Event Signal1/1 -> MATLAB Function/3(PickStdDev)
  eachPickMean/1 -> Timed to Event Signal/1
  Timed to Event Signal/1 -> MATLAB Function/2(PickMean)
  TravelTime/1 -> Timed to Event Signal2/1
  Timed to Event Signal2/1 -> Add/2
  connections:
  Get Attribute/RConn1 -- Single Server/LConn1
  IN_Order/RConn1 -- Get Attribute/LConn1
  OUT_Order/RConn1 -- Single Server/RConn1

== system ProcessFlowRateModel_symbiotic/Shipping/Workstation/Shipping/Process ==
  FIFO Queue : FIFOQueue  Capacity=inf
  N-Server : NServer  NumberOfServers=inf  ServiceTimeFrom=Signal port t
  ProcessTime : EventBasedRandomNumber  Distribution=Arbitrary discrete  minUnif=1  meanNorm=5  minUnid=29.9  maxUnid=30  numValueUnid=1  valueVecDisc=[0 30]  probVecDisc=[0 1]
  Job_OUT : PMIOPort  Port=1  Side=Right
  Job_IN : PMIOPort  Port=2  Side=Left
  wires:
  ProcessTime/1 -> N-Server/1
  connections:
  FIFO Queue/RConn1 -- N-Server/LConn1
  Job_OUT/RConn1 -- N-Server/RConn1
  Job_IN/RConn1 -- FIFO Queue/LConn1

== matlab function PickCartonFromPalletStore_2/Workstation/CartonPick/Pick_CycleTime/MATLAB Function ==
  data: Quantity input double; PickCycleTime output double; PickMean input double; PickStdDev input double
function PickCycleTime = fcn(Quantity,  PickMean, PickStdDev)
%#codegen

coder.extrinsic('normrnd');
PickCycleTime = zeros(1, 'double');

Pick_Mean = Quantity*PickMean;
Pick_StdDev =Quantity*PickStdDev;

PickCycleTime = normrnd(Pick_Mean, sqrt(Pick_StdDev));

== matlab function Subsystem1/Pick_CycleTime/MATLAB Function ==
  data: Quantity input double; PickCycleTime output double; PickMean input double; PickStdDev input double
function PickCycleTime = fcn(Quantity,  PickMean, PickStdDev)
%#codegen

coder.extrinsic('normrnd');
PickCycleTime = zeros(1, 'double');

Pick_Mean = Quantity*PickMean;
Pick_StdDev =Quantity*PickStdDev;

PickCycleTime = normrnd(Pick_Mean, sqrt(Pick_StdDev));

end

== matlab function Subsystem/Pick_CycleTime/MATLAB Function ==
  data: Quantity input double; PickCycleTime output double; PickMean input double; PickStdDev input double
function PickCycleTime = fcn(Quantity,  PickMean, PickStdDev)
%#codegen

coder.extrinsic('normrnd');
PickCycleTime = zeros(1, 'double');

Pick_Mean = Quantity*PickMean;
Pick_StdDev =Quantity*PickStdDev;

PickCycleTime = normrnd(Pick_Mean, sqrt(Pick_StdDev));

end

== matlab function Subsystem1/Unblock_Selector ==
  data: en output double; wip input double; n input double
function en = fcn(wip, n)

aVarTruthTableCondition_1 = false;
aVarTruthTableCondition_2 = false;


% Server is available;

aVarTruthTableCondition_1 = logical(n == 0);

% Symbiotic is ready;

aVarTruthTableCondition_2 = logical(wip == 1);

if (aVarTruthTableCondition_1 && aVarTruthTableCondition_2)
    aFcnTruthTableAction_1();
elseif (~aVarTruthTableCondition_1 && ~aVarTruthTableCondition_2)
    aFcnTruthTableAction_2();
elseif (aVarTruthTableCondition_1 && ~aVarTruthTableCondition_2)
    aFcnTruthTableAction_2();
else % Default
    aFcnTruthTableAction_2();
end

function aFcnTruthTableAction_1()

% Release Selector

en = 1;

function aFcnTruthTableAction_2()

% Block Selector

en = 0;

== matlab function Subsystem2/Pick_CycleTime/MATLAB Function ==
  data: Quantity input double; PickCycleTime output double; PickMean input double; PickStdDev input double
function PickCycleTime = fcn(Quantity,  PickMean, PickStdDev)
%#codegen

coder.extrinsic('normrnd');
PickCycleTime = zeros(1, 'double');

Pick_Mean = Quantity*PickMean;
Pick_StdDev =Quantity*PickStdDev;

PickCycleTime = normrnd(Pick_Mean, sqrt(Pick_StdDev));

end

== matlab function Subsystem2/Unblock_Selector ==
  data: en output double; wip input double; n input double
function en = fcn(wip, n)

aVarTruthTableCondition_1 = false;
aVarTruthTableCondition_2 = false;


% Server is available;

aVarTruthTableCondition_1 = logical(n == 0);

% Symbiotic is ready;

aVarTruthTableCondition_2 = logical(wip == 1);

if (aVarTruthTableCondition_1 && aVarTruthTableCondition_2)
    aFcnTruthTableAction_1();
elseif (~aVarTruthTableCondition_1 && ~aVarTruthTableCondition_2)
    aFcnTruthTableAction_2();
elseif (aVarTruthTableCondition_1 && ~aVarTruthTableCondition_2)
    aFcnTruthTableAction_2();
else % Default
    aFcnTruthTableAction_2();
end

function aFcnTruthTableAction_1()

% Release Selector

en = 1;

function aFcnTruthTableAction_2()

% Block Selector

en = 0;

== matlab function Subsystem3/Pick_CycleTime/MATLAB Function ==
  data: Quantity input double; PickCycleTime output double; PickMean input double; PickStdDev input double
function PickCycleTime = fcn(Quantity,  PickMean, PickStdDev)
%#codegen

coder.extrinsic('normrnd');
PickCycleTime = zeros(1, 'double');

Pick_Mean = Quantity*PickMean;
Pick_StdDev =Quantity*PickStdDev;

PickCycleTime = normrnd(Pick_Mean, sqrt(Pick_StdDev));

end

== matlab function Subsystem/Unblock_Selector ==
  data: en output double; wip input double; n input double
function en = fcn(wip, n)

aVarTruthTableCondition_1 = false;
aVarTruthTableCondition_2 = false;


% Server is available;

aVarTruthTableCondition_1 = logical(n == 0);

% Symbiotic is ready;

aVarTruthTableCondition_2 = logical(wip == 1);

if (aVarTruthTableCondition_1 && aVarTruthTableCondition_2)
    aFcnTruthTableAction_1();
elseif (~aVarTruthTableCondition_1 && ~aVarTruthTableCondition_2)
    aFcnTruthTableAction_2();
elseif (aVarTruthTableCondition_1 && ~aVarTruthTableCondition_2)
    aFcnTruthTableAction_2();
else % Default
    aFcnTruthTableAction_2();
end

function aFcnTruthTableAction_1()

% Release Selector

en = 1;

function aFcnTruthTableAction_2()

% Block Selector

en = 0;

== matlab function Subsystem3/Unblock_Selector ==
  data: en output double; wip input double; n input double
function en = fcn(wip, n)

aVarTruthTableCondition_1 = false;
aVarTruthTableCondition_2 = false;


% Server is available;

aVarTruthTableCondition_1 = logical(n == 0);

% Symbiotic is ready;

aVarTruthTableCondition_2 = logical(wip == 1);

if (aVarTruthTableCondition_1 && aVarTruthTableCondition_2)
    aFcnTruthTableAction_1();
elseif (~aVarTruthTableCondition_1 && ~aVarTruthTableCondition_2)
    aFcnTruthTableAction_2();
elseif (aVarTruthTableCondition_1 && ~aVarTruthTableCondition_2)
    aFcnTruthTableAction_2();
else % Default
    aFcnTruthTableAction_2();
end

function aFcnTruthTableAction_1()

% Release Selector

en = 1;

function aFcnTruthTableAction_2()

% Block Selector

en = 0;

== matlab function Subsystem4/Pick_CycleTime/MATLAB Function ==
  data: Quantity input double; PickCycleTime output double; PickMean input double; PickStdDev input double
function PickCycleTime = fcn(Quantity,  PickMean, PickStdDev)
%#codegen

coder.extrinsic('normrnd');
PickCycleTime = zeros(1, 'double');

Pick_Mean = Quantity*PickMean;
Pick_StdDev =Quantity*PickStdDev;

PickCycleTime = normrnd(Pick_Mean, sqrt(Pick_StdDev));

end

== matlab function PickCartonFromPalletStore_1/Workstation/CartonPick/Pick_CycleTime/MATLAB Function ==
  data: Quantity input double; PickCycleTime output double; PickMean input double; PickStdDev input double
function PickCycleTime = fcn(Quantity,  PickMean, PickStdDev)
%#codegen

coder.extrinsic('normrnd');
PickCycleTime = zeros(1, 'double');

Pick_Mean = Quantity*PickMean;
Pick_StdDev =Quantity*PickStdDev;

PickCycleTime = normrnd(Pick_Mean, sqrt(Pick_StdDev));

== matlab function Subsystem4/Unblock_Selector ==
  data: en output double; wip input double; n input double
function en = fcn(wip, n)

aVarTruthTableCondition_1 = false;
aVarTruthTableCondition_2 = false;


% Server is available;

aVarTruthTableCondition_1 = logical(n == 0);

% Symbiotic is ready;

aVarTruthTableCondition_2 = logical(wip == 1);

if (aVarTruthTableCondition_1 && aVarTruthTableCondition_2)
    aFcnTruthTableAction_1();
elseif (~aVarTruthTableCondition_1 && ~aVarTruthTableCondition_2)
    aFcnTruthTableAction_2();
elseif (aVarTruthTableCondition_1 && ~aVarTruthTableCondition_2)
    aFcnTruthTableAction_2();
else % Default
    aFcnTruthTableAction_2();
end

function aFcnTruthTableAction_1()

% Release Selector

en = 1;

function aFcnTruthTableAction_2()

% Block Selector

en = 0;

== matlab function Subsystem5/Pick_CycleTime/MATLAB Function ==
  data: Quantity input double; PickCycleTime output double; PickMean input double; PickStdDev input double
function PickCycleTime = fcn(Quantity,  PickMean, PickStdDev)
%#codegen

coder.extrinsic('normrnd');
PickCycleTime = zeros(1, 'double');

Pick_Mean = Quantity*PickMean;
Pick_StdDev =Quantity*PickStdDev;

PickCycleTime = normrnd(Pick_Mean, sqrt(Pick_StdDev));

end

== matlab function Subsystem5/Unblock_Selector ==
  data: en output double; wip input double; n input double
function en = fcn(wip, n)

aVarTruthTableCondition_1 = false;
aVarTruthTableCondition_2 = false;


% Server is available;

aVarTruthTableCondition_1 = logical(n == 0);

% Symbiotic is ready;

aVarTruthTableCondition_2 = logical(wip == 1);

if (aVarTruthTableCondition_1 && aVarTruthTableCondition_2)
    aFcnTruthTableAction_1();
elseif (~aVarTruthTableCondition_1 && ~aVarTruthTableCondition_2)
    aFcnTruthTableAction_2();
elseif (aVarTruthTableCondition_1 && ~aVarTruthTableCondition_2)
    aFcnTruthTableAction_2();
else % Default
    aFcnTruthTableAction_2();
end

function aFcnTruthTableAction_1()

% Release Selector

en = 1;

function aFcnTruthTableAction_2()

% Block Selector

en = 0;
